simulink model "matlabmodel"  (R2025b)
settings: Solver=ode4  StartTime=0.0  StopTime=inf  FixedStep=0.1  RelTol=1e-3
libraries: simulink x3
settings Model: Creator=Pragati-TRN0433  LastModifiedBy=Pragati-TRN0433

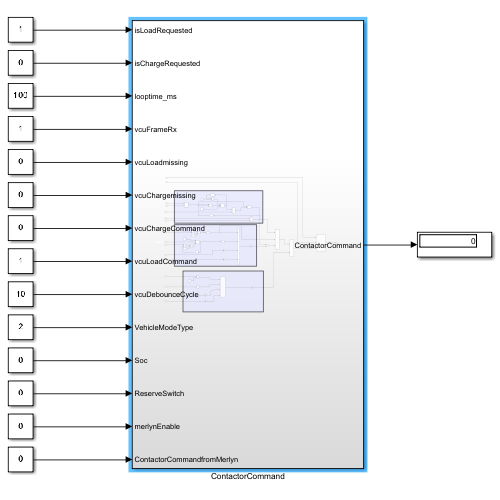
[thumbnail: Simulink's stored preview of the top-level diagram]
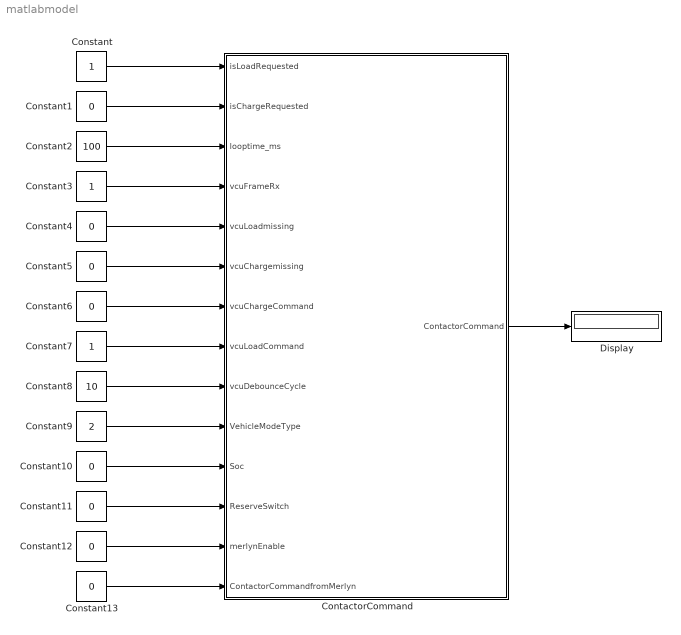
== system matlabmodel ==
  Constant : Constant
  Constant{1,4..6,10..13} (8 alike) : Constant  Value=0
  Constant2 : Constant  Value=100  OutDataTypeStr=uint32
  Constant3 : Constant
  Constant7 : Constant
  Constant8 : Constant  Value=10
  Constant9 : Constant  Value=2
  ContactorCommand : Subsystem
  Display : Display
  wires:
  Constant/1 -> ContactorCommand/1(isLoadRequested)
  Constant2/1 -> ContactorCommand/3(looptime_ms)
  Constant4/1 -> ContactorCommand/5(vcuLoadmissing)
  Constant5/1 -> ContactorCommand/6(vcuChargemissing)
  Constant3/1 -> ContactorCommand/4(vcuFrameRx)
  Constant1/1 -> ContactorCommand/2(isChargeRequested)
  Constant6/1 -> ContactorCommand/7(vcuChargeCommand)
  Constant7/1 -> ContactorCommand/8(vcuLoadCommand)
  Constant8/1 -> ContactorCommand/9(vcuDebounceCycle)
  Constant9/1 -> ContactorCommand/10(VehicleModeType)
  Constant10/1 -> ContactorCommand/11(Soc)
  Constant11/1 -> ContactorCommand/12(ReserveSwitch)
  Constant12/1 -> ContactorCommand/13(merlynEnable)
  Constant13/1 -> ContactorCommand/14(ContactorCommandfromMerlyn)
  ContactorCommand/1(ContactorCommand) -> Display/1

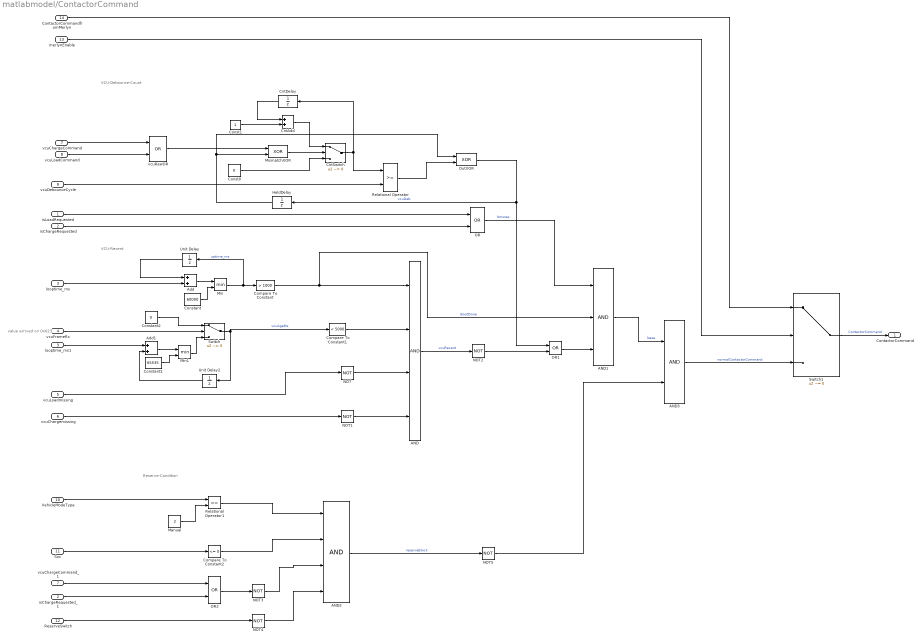
== system matlabmodel/ContactorCommand ==
  note: VCU-Debounce-Count
  note: VCU-Recent
  note: Reserve-Condition
  note: value arrived on 0x623
  isLoadRequested : Inport
  isChargeRequested : Inport  Port=2
  looptime_ms : Inport  Port=3  OutDataTypeStr=uint32
  vcuFrameRx : Inport  Port=4
  vcuLoadmissing : Inport  Port=5
  vcuChargemissing : Inport  Port=6
  vcuChargeCommand : Inport  Port=7
  vcuLoadCommand : Inport  Port=8
  vcuDebounceCycle : Inport  Port=9
  VehicleModeType : Inport  Port=10
  Soc : Inport  Port=11
  ReserveSwitch : Inport  Port=12
  merlynEnable : Inport  Port=13
  ContactorCommandfromMerlyn : Inport  Port=14
  AND : Logic  Inputs=4  IconShape=distinctive  AllPortsSameDT=off  OutDataTypeStr=boolean
  AND1 : Logic  Inputs=3  AllPortsSameDT=off  OutDataTypeStr=boolean
  AND2 : Logic  Inputs=4  AllPortsSameDT=off  OutDataTypeStr=boolean
  AND3 : Logic  AllPortsSameDT=off  OutDataTypeStr=boolean
  Add : Sum  OutDataTypeStr=uint32
  Add1 : Sum
  CntAdd : Sum  OutDataTypeStr=uint8  SaturateOnIntegerOverflow=on
  CntDelay : UnitDelay  SampleTime=-1  HasFrameUpgradeWarning=on
  CntSwitch : Switch  Criteria=u2 ~= 0  SaturateOnIntegerOverflow=off  InputSameDT=off
  Compare To Constant : simulink/Logic and Bit Operations/Compare To Constant  relop=>  const=1000  OutDataTypeStr=boolean
  Compare To Constant1 : simulink/Logic and Bit Operations/Compare To Constant  relop=<  const=5000  OutDataTypeStr=boolean
  Compare To Constant2 : simulink/Logic and Bit Operations/Compare To Constant  relop=<=  const=0  OutDataTypeStr=boolean
  Const0 : Constant  Value=0  OutDataTypeStr=uint8
  Const1 : Constant  OutDataTypeStr=uint8
  Constant : Constant  Value=60000  OutDataTypeStr=uint32
  Constant1 : Constant  Value=65535  OutDataTypeStr=uint32
  Constant2 : Constant  Value=0
  HeldDelay : UnitDelay  SampleTime=-1  HasFrameUpgradeWarning=on
  Manual : Constant  Value=2
  Min : MinMax  Inputs=2  OutDataTypeStr=uint32
  Min1 : MinMax  Inputs=2
  MismatchXOR : Logic  Operator=XOR  AllPortsSameDT=off  OutDataTypeStr=boolean
  NOT{,1..5} (6 alike) : Logic  Operator=NOT  IconShape=distinctive  AllPortsSameDT=off  OutDataTypeStr=boolean
  OR : Logic  Operator=OR  AllPortsSameDT=off  OutDataTypeStr=boolean
  OR1 : Logic  Operator=OR  AllPortsSameDT=off  OutDataTypeStr=boolean
  OR2 : Logic  Operator=OR  AllPortsSameDT=off  OutDataTypeStr=boolean
  OutXOR : Logic  Operator=XOR  AllPortsSameDT=off  OutDataTypeStr=boolean
  Relational Operator : RelationalOperator  OutDataTypeStr=boolean  RndMeth=Simplest  InputSameDT=off
  Relational Operator1 : RelationalOperator  Operator===  OutDataTypeStr=boolean  RndMeth=Simplest  InputSameDT=off
  Switch : Switch  Criteria=u2 ~= 0  SaturateOnIntegerOverflow=off  InputSameDT=off
  Switch1 : Switch  Criteria=u2 ~= 0  SaturateOnIntegerOverflow=off  InputSameDT=off
  Unit Delay : UnitDelay  SampleTime=-1  HasFrameUpgradeWarning=on
  Unit Delay2 : UnitDelay  InitialCondition=65535  SampleTime=-1  HasFrameUpgradeWarning=on
  isChargeRequested_1 : InportShadow  Port=2
  looptime_ms1 : InportShadow  Port=3  OutDataTypeStr=uint32
  vcuChargeCommand_1 : InportShadow  Port=7
  vcuRawOR : Logic  Operator=OR  AllPortsSameDT=off  OutDataTypeStr=boolean
  ContactorCommand : Outport
  wires:
  VehicleModeType/1 -> Relational Operator1/1
  Manual/1 -> Relational Operator1/2
  Min1/1 -> Switch/3
  NOT2/1 -> OR1/2
  Add/1 -> Min/1
  Constant1/1 -> Min1/2
  CntSwitch/1 -> Relational Operator/1, CntDelay/1
  NOT4/1 -> AND2/4
  isChargeRequested/1 -> OR/2
  isChargeRequested_1/1 -> OR2/2
  ReserveSwitch/1 -> NOT4/1
  vcuLoadmissing/1 -> NOT/1
  vcuChargeCommand_1/1 -> OR2/1
  AND/1 -> NOT2/1  "vcuRecent"
  NOT5/1 -> AND3/2
  Constant/1 -> Min/2
  Min/1 -> Unit Delay/1, Compare To Constant/1  "uptime_ms"
  merlynEnable/1 -> Switch1/2
  vcuDebounceCycle/1 -> Relational Operator/2
  OR2/1 -> NOT3/1
  vcuChargemissing/1 -> NOT1/1
  Unit Delay2/1 -> Add1/2
  Compare To Constant2/1 -> AND2/2
  looptime_ms/1 -> Add/2
  CntAdd/1 -> CntSwitch/1
  AND1/1 -> AND3/1  "base"
  AND2/1 -> NOT5/1  "reserveBlock"
  ContactorCommandfromMerlyn/1 -> Switch1/1
  OutXOR/1 -> OR1/1, HeldDelay/1  "vcuDeb"
  Const1/1 -> CntAdd/2
  Compare To Constant/1 -> AND1/2, AND/1  "BootDone"
  HeldDelay/1 -> OutXOR/1, MismatchXOR/2
  NOT3/1 -> AND2/3
  NOT/1 -> AND/3
  isLoadRequested/1 -> OR/1
  Switch/1 -> Unit Delay2/1, Compare To Constant1/1  "vcuAgeMs"
  Add1/1 -> Min1/1
  AND3/1 -> Switch1/3  "normalContactorCommand"
  CntDelay/1 -> CntAdd/1
  Soc/1 -> Compare To Constant2/1
  OR/1 -> AND1/1  "bmsreq"
  vcuChargeCommand/1 -> vcuRawOR/1
  Unit Delay/1 -> Add/1
  Constant2/1 -> Switch/1
  Compare To Constant1/1 -> AND/2
  MismatchXOR/1 -> CntSwitch/2
  Const0/1 -> CntSwitch/3
  vcuFrameRx/1 -> Switch/2
  vcuRawOR/1 -> MismatchXOR/1
  OR1/1 -> AND1/3
  NOT1/1 -> AND/4
  Relational Operator1/1 -> AND2/1
  Relational Operator/1 -> OutXOR/2
  vcuLoadCommand/1 -> vcuRawOR/2
  Switch1/1 -> ContactorCommand/1  "ContactorCommand"
  looptime_ms1/1 -> Add1/1
